simulink model "ForwardMotor_ForceMoment"  (R2025a)
settings: Solver=VariableStepAuto  StartTime=0.0  StopTime=10.0  RelTol=1e-3
undefined symbols (not defined in the file or in its folder): FM1_POSITION, FM2_POSITION
settings Model: Creator=Ayush_S  LastModifiedBy=Ayush_S

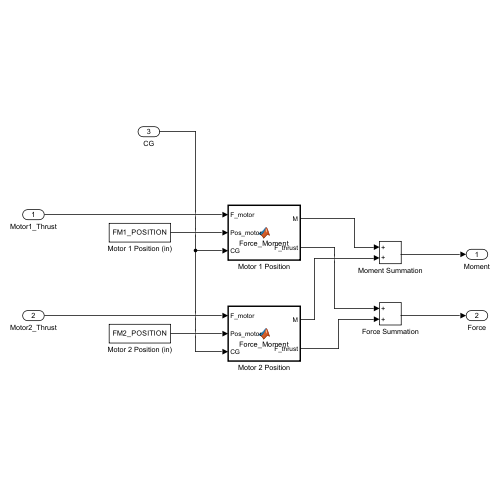
[thumbnail: Simulink's stored preview of the top-level diagram]
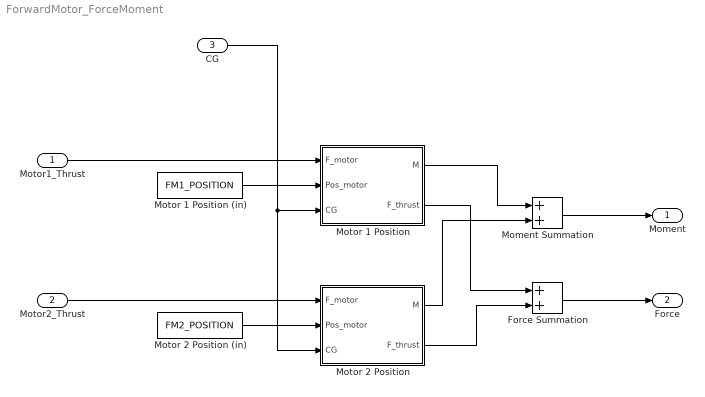
== system ForwardMotor_ForceMoment ==
  Motor1_Thrust : Inport
  Motor2_Thrust : Inport  Port=2
  CG : Inport  Port=3
  Force Summation : Sum
  Moment Summation : Sum
  Motor 1 Position : MATLAB Function  TreatAsAtomicUnit=on
  Motor 1 Position (in) : Constant  Value=FM1_POSITION  VectorParams1D=off
  Motor 2 Position : MATLAB Function  TreatAsAtomicUnit=on
  Motor 2 Position (in) : Constant  Value=FM2_POSITION  VectorParams1D=off
  Moment : Outport
  Force : Outport  Port=2
  wires:
  CG/1 -> Motor 1 Position/3(CG), Motor 2 Position/3(CG)
  Motor 2 Position (in)/1 -> Motor 2 Position/2(Pos_motor)
  Motor 1 Position (in)/1 -> Motor 1 Position/2(Pos_motor)
  Motor2_Thrust/1 -> Motor 2 Position/1(F_motor)
  Motor1_Thrust/1 -> Motor 1 Position/1(F_motor)
  Motor 1 Position/2(F_thrust) -> Force Summation/1
  Motor 2 Position/2(F_thrust) -> Force Summation/2
  Motor 2 Position/1(M) -> Moment Summation/2
  Force Summation/1 -> Force/1
  Moment Summation/1 -> Moment/1
  Motor 1 Position/1(M) -> Moment Summation/1

== matlab function ForwardMotor_ForceMoment/Motor 2 Position ==
  data: F_motor input; M output; Pos_motor input; CG input; F_thrust output
function [M,F_thrust] = Force_Moment(F_motor, Pos_motor, CG) 
    F_thrust = F_motor .* [1 0 0]; % gets x variable of thrust coordinate
    
    R = Pos_motor - CG; % Motor position vector, CG to motor 
        
    Moment = cross(R, F_thrust);

M = Moment;

== matlab function ForwardMotor_ForceMoment/Motor 1 Position ==
  data: F_motor input; M output; Pos_motor input; CG input; F_thrust output
function [M,F_thrust] = Force_Moment(F_motor, Pos_motor, CG) 
    F_thrust = F_motor .* [1 0 0]; % gets x variable of thrust coordinate
    
    R = Pos_motor - CG; % Motor position vector, CG to motor 
        
    Moment = cross(R, F_thrust);

M = Moment;
